simulink model "CoefNormalForce_TestModel"  (R2014a)
settings: Solver=ode45  StartTime=0.0  StopTime=10.0  RelTol=1e-3
libraries: rocket_angular_flight_library x2
settings Model: Creator=scorpii  LastModifiedBy=scorpii

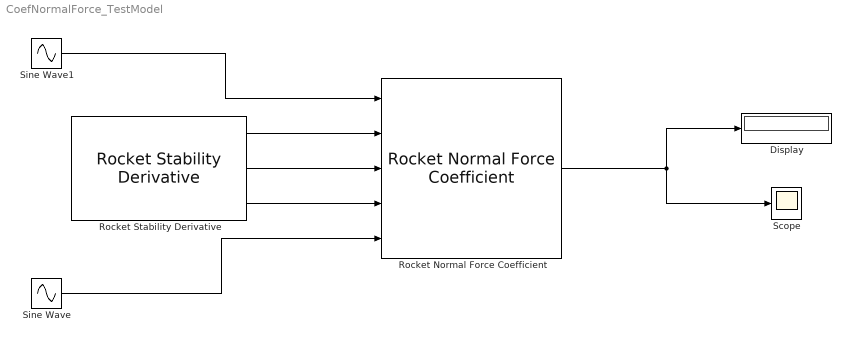
== system CoefNormalForce_TestModel ==
  Display : Display
  Rocket Normal Force Coefficient : rocket_angular_flight_library/Rocket Normal Force Coefficient
  Rocket Stability Derivative : rocket_angular_flight_library/Rocket Stability Derivative
  Scope : Scope
  Sine Wave : Sin  Phase=pi  SampleTime=0
  Sine Wave1 : Sin  SampleTime=0
  wires:
  Rocket Stability Derivative/1 -> Rocket Normal Force Coefficient/2
  Rocket Stability Derivative/2 -> Rocket Normal Force Coefficient/3
  Rocket Stability Derivative/3 -> Rocket Normal Force Coefficient/4
  Sine Wave/1 -> Rocket Normal Force Coefficient/5
  Sine Wave1/1 -> Rocket Normal Force Coefficient/1
  Rocket Normal Force Coefficient/1 -> Scope/1, Display/1
